simulink model "Project_Part2"  (R2024b)
settings: Solver=VariableStepAuto  StartTime=0.0  StopTime=3  RelTol=1e-3
libraries: shared6dof x1
settings Model: Creator=arnoldpretorius  LastModifiedBy=arnoldpretorius

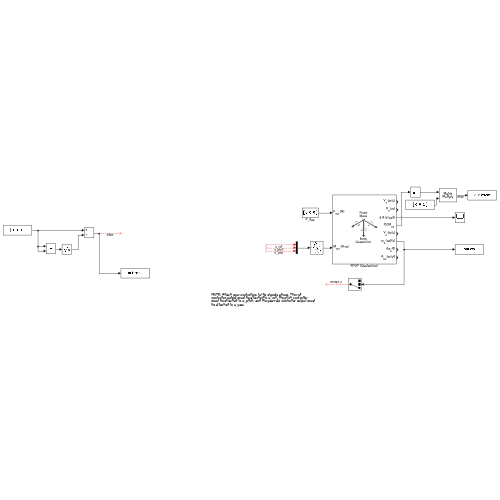
[thumbnail: Simulink's stored preview of the top-level diagram]
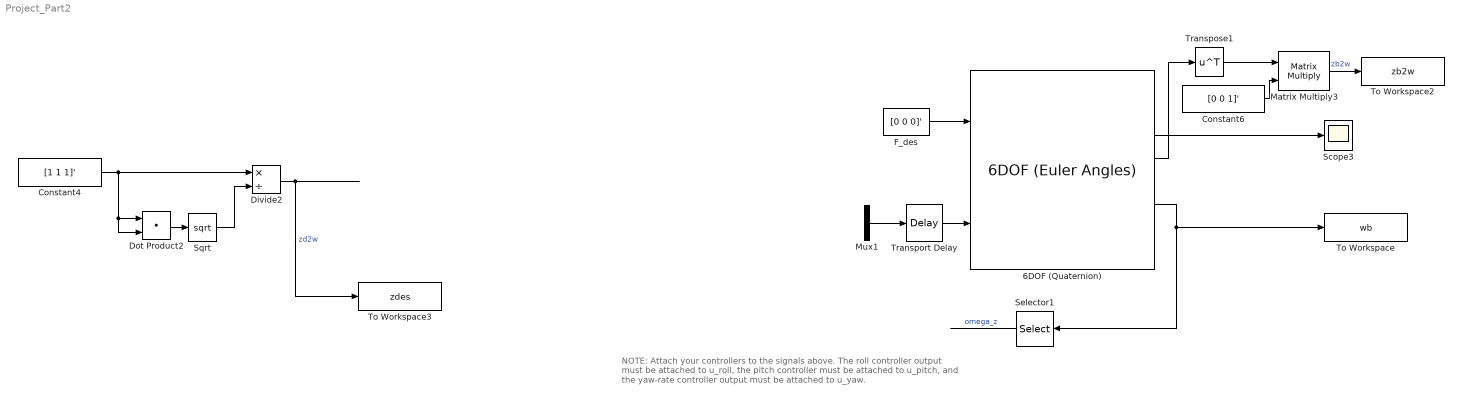
== system Project_Part2 ==
  note: NOTE: Attach your controllers to the signals above. The roll controller output must be attached to u_roll, the pitch controller must be attached to u_pitch, and the yaw-rate controller output must be attached to u_yaw.
  6DOF (Quaternion) : shared6dof/6DOF (Euler Angles)  units=Metric (MKS)  mtype=Fixed  rep=Quaternion  xme_0=[0 0 0]  Vm_0=[0 0 0]  eul_0=[0 0 0]  pm_0=[0 0 0]  mass_0=1.0  mass_e=0.5  mass_f=2.0  inertia=diag([2e-3,2.3e-3,4.5e-3])  inertia_e=eye(3)  inertia_f=2*eye(3)  k_quat=1.0  vre_flag=on  abi_flag=off  aMode=0  xme_statename=''  Vm_statename=''  eul_statename=''  quat_statename=''  pm_statename=''  mass_statename=''
      settings: LibrarySourceBlock=aerolib6dof2/6DOF (Quaternion)
  Constant4 : Constant  Value=[1 1 1]'
  Constant6 : Constant  Value=[0 0 1]'
  Divide2 : Product  Inputs=*/
  Dot Product2 : DotProduct  OutDataTypeStr=Inherit: Inherit via internal rule
  F_des : Constant  Value=[0 0 0]'
  Matrix Multiply3 : Product  Multiplication=Matrix(*)
  Mux1 : Mux  Inputs=3
  Scope3 : Scope
  Selector1 : Selector  InputPortWidth=3  IndexOptions=Index vector (dialog)  Indices=[3]  OutputSizes=1
  Sqrt : Sqrt
  To Workspace : ToWorkspace  VariableName=wb  SaveFormat=Timeseries  SampleTime=-1
  To Workspace2 : ToWorkspace  VariableName=zb2w  SaveFormat=Timeseries  SampleTime=-1
  To Workspace3 : ToWorkspace  VariableName=zdes  SaveFormat=Timeseries  SampleTime=-1
  Transport Delay : TransportDelay  DelayTime=0.005
  Transpose1 : Math  Operator=transpose
  wires:
  Constant4/1 -> Divide2/1, Dot Product2/2, Dot Product2/1
  6DOF (Quaternion)/3 -> Scope3/1
  6DOF (Quaternion)/4 -> Transpose1/1
  Divide2/1 -> To Workspace3/1  "zd2w"
  Matrix Multiply3/1 -> To Workspace2/1  "zb2w"
  Transpose1/1 -> Matrix Multiply3/1
  Constant6/1 -> Matrix Multiply3/2
  F_des/1 -> 6DOF (Quaternion)/1
  Transport Delay/1 -> 6DOF (Quaternion)/2
  Mux1/1 -> Transport Delay/1
  6DOF (Quaternion)/6 -> To Workspace/1, Selector1/1
  Dot Product2/1 -> Sqrt/1
  Sqrt/1 -> Divide2/2
  Selector1/1 -> ?  "omega_z"
  ? -> Mux1/1  "u_roll"
  ? -> Mux1/2  "u_pitch"
  ? -> Mux1/3  "u_yaw"
